simulink subsystem "Subsystem_Weather_BAv02"  (R2022b)
settings: Solver=VariableStepAuto  StartTime=0.0  StopTime=10.0  RelTol=1e-3
undefined symbols (not defined in the file): weatherSim
settings Model: Creator=giaco  LastModifiedBy=giaco

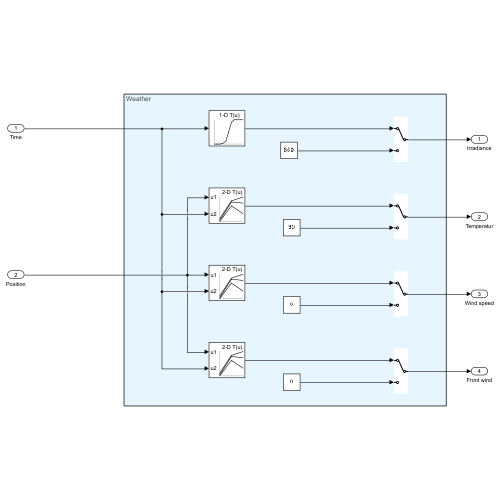
[thumbnail: Simulink's stored preview of the top-level diagram]
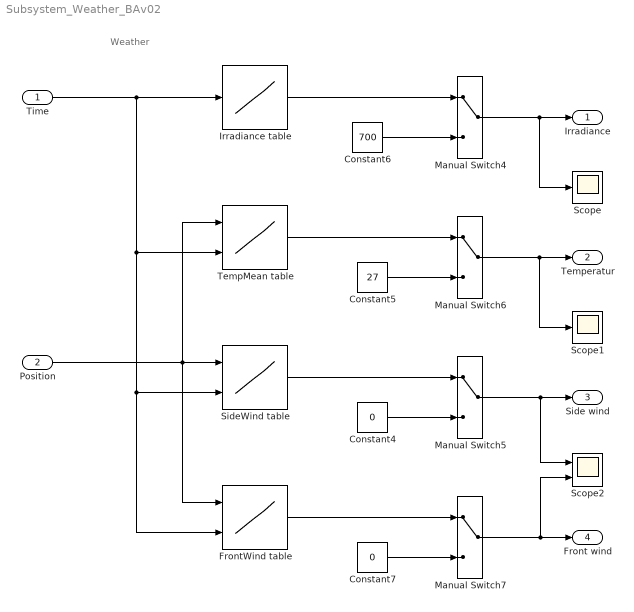
== system Subsystem_Weather_BAv02 ==
  note: Weather
  Time : Inport
  Position : Inport  Port=2
  Constant4 : Constant  Value=0
  Constant5 : Constant  Value=27
  Constant6 : Constant  Value=700
  Constant7 : Constant  Value=0
  FrontWind table : Lookup_n-D  BreakpointsForDimension1=weatherSim.wind.dist(1:end-1)  BreakpointsForDimension2=weatherSim.wind.timeSec  Table=weatherSim.wind.frontWind  InternalRulePriority=Speed  RndMeth=Simplest
      settings: InputPortMap=u0,u1
  Irradiance table : Lookup_n-D  NumberOfTableDimensions=1  BreakpointsForDimension1=weatherSim.irradiance.timeSec  Table=weatherSim.irradiance.GtotalSec  InternalRulePriority=Speed  RndMeth=Simplest
  Manual Switch{4..7} (4 alike) : ManualSwitch
  Scope : Scope
  Scope1 : Scope
  Scope2 : Scope  NumInputPorts=2
  SideWind table : Lookup_n-D  BreakpointsForDimension1=weatherSim.wind.dist(1:end-1)  BreakpointsForDimension2=weatherSim.wind.timeSec  Table=weatherSim.wind.sideWind  InternalRulePriority=Speed  RndMeth=Simplest
      settings: InputPortMap=u0,u1
  TempMean table : Lookup_n-D  BreakpointsForDimension1=weatherSim.temperature.dist  BreakpointsForDimension2=weatherSim.temperature.timeSec  Table=weatherSim.temperature.tempMean  InternalRulePriority=Speed  RndMeth=Simplest
      settings: InputPortMap=u0,u1
  Irradiance : Outport
  Temperatur : Outport  Port=2
  Side wind : Outport  Port=3
  Front wind : Outport  Port=4
  wires:
  Constant5/1 -> Manual Switch6/2
  FrontWind table/1 -> Manual Switch7/1
  Irradiance table/1 -> Manual Switch4/1
  Manual Switch4/1 -> Irradiance/1, Scope/1
  Constant6/1 -> Manual Switch4/2
  TempMean table/1 -> Manual Switch6/1
  Manual Switch7/1 -> Front wind/1, Scope2/2
  SideWind table/1 -> Manual Switch5/1
  Constant4/1 -> Manual Switch5/2
  Constant7/1 -> Manual Switch7/2
  Manual Switch6/1 -> Temperatur/1, Scope1/1
  Manual Switch5/1 -> Side wind/1, Scope2/1
  Time/1 -> TempMean table/2, SideWind table/2, FrontWind table/2, Irradiance table/1
  Position/1 -> FrontWind table/1, SideWind table/1, TempMean table/1
